simulink model "hand_nofeedback"  (R2013a)
settings: Solver=ode45  StartTime=0.0  StopTime=10.0  MaxStep=1  RelTol=1e-3
values from neighbouring files (symbols this model uses):
  m = size(t,2)    [ff.m]    (also in findGradientPend.m; interpolate.m = min(dss,[],2))
  s = @(t) [sqrt(l^2 - p(2,t).^2) + p(1,t) ; 0]    [basic.m]    (also in evaluate.m = model(p); f.m = [[l;0] zeros(2,n-1)]; ff.m = [[l;0] zeros(2,m-1)]; model.m = zeros(2,1))
libraries: mblibv1 x14, simulink x5
settings Model: Creator=annie  LastModifiedBy=simplehands
settings DataIOCC: SignalLoggingSaveFormat=ModelDataLogs
settings OptimizationCC: ExpressionDepthLimit=2147483647
settings DebuggingCC: FcnCallInpInsideContextMsg=EnableAllAsWarning
settings SimMechanicsCC: VisDuringSimulation=on

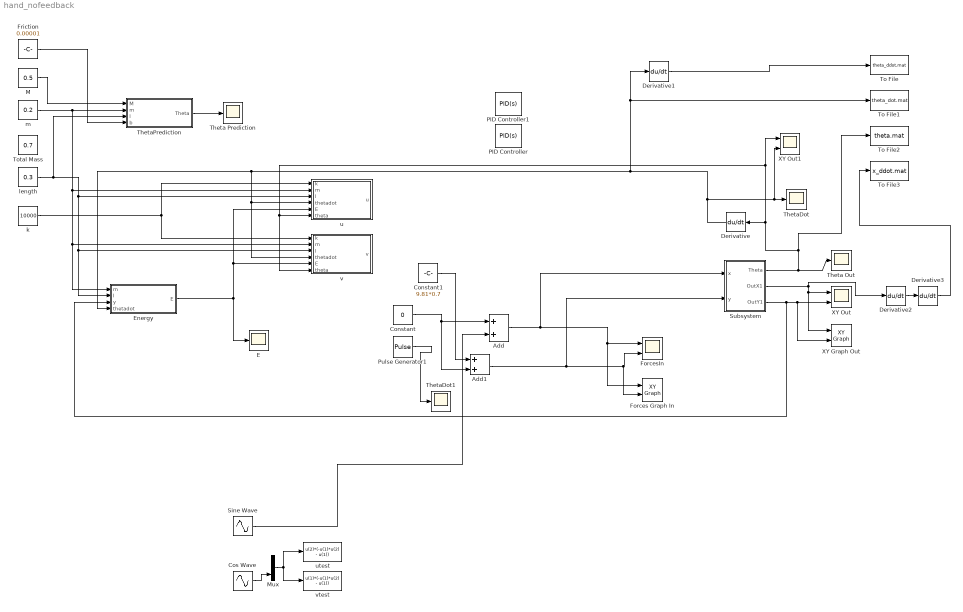
== system hand_nofeedback ==
  Add : Sum
  Add1 : Sum
  Constant : Constant  Value=0
  Constant1 : Constant  Value=9.81*0.7
  Cos Wave : Sin  Phase=pi/2  SampleTime=0
  Derivative{,1..3} (4 alike) : Derivative
  E : Scope
      settings: TimeRange=10  YMin=-0.025  YMax=0.0025  SaveName=ScopeData5
  Energy : Subsystem
  Forces Graph In : simulink/Sinks/XY Graph  xmin=-1  xmax=1  ymin=-1  ymax=1  st=-1
  ForcesIn : Scope  NumInputPorts=2
      settings: TimeRange=10  YMin=-0.1~-0.1  YMax=0.25~0.25  SaveName=ScopeData2
  Friction : Constant  Value=0.00001
  M : Constant  Value=0.5
  Mux : Mux  Inputs=2
  PID Controller : simulink/Continuous/PID Controller  Controller=PID  TimeDomain=Continuous-time  SampleTime=1  IntegratorMethod=Forward Euler  FilterMethod=Forward Euler  Form=Parallel  P=1  I=1  D=0  N=100  InitialConditionSource=internal  InitialConditionForIntegrator=0  InitialConditionForFilter=0  ExternalReset=none  LimitOutput=off  UpperSaturationLimit=inf  LowerSaturationLimit=-inf  LinearizeAsGain=on  AntiWindupMode=none  Kb=1  TrackingMode=off  Kt=1  PParamMin=[]  PParamMax=[]  IParamMin=[]  IParamMax=[]  DParamMin=[]  DParamMax=[]  NParamMin=[]  NParamMax=[]  KbParamMin=[]  KbParamMax=[]  KtParamMin=[]  KtParamMax=[]  POutMin=[]  POutMax=[]  IOutMin=[]  IOutMax=[]  DOutMin=[]  DOutMax=[]  NOutMin=[]  NOutMax=[]  KbOutMin=[]  KbOutMax=[]  KtOutMin=[]  KtOutMax=[]  IntegratorOutMin=[]  IntegratorOutMax=[]  FilterOutMin=[]  FilterOutMax=[]  SumOutMin=[]  SumOutMax=[]  SumI1OutMin=[]  SumI1OutMax=[]  SumI2OutMin=[]  SumI2OutMax=[]  SumI3OutMin=[]  SumI3OutMax=[]  SumDOutMin=[]  SumDOutMax=[]  SaturationOutMin=[]  SaturationOutMax=[]  IntegratorContinuousStateAttributes=''  IntegratorStateMustResolveToSignalObject=off  IntegratorRTWStateStorageClass=Auto  FilterContinuousStateAttributes=''  FilterStateMustResolveToSignalObject=off  FilterRTWStateStorageClass=Auto
  PID Controller1 : simulink/Continuous/PID Controller  Controller=PID  TimeDomain=Continuous-time  SampleTime=1  IntegratorMethod=Forward Euler  FilterMethod=Forward Euler  Form=Parallel  P=1  I=1  D=0  N=100  InitialConditionSource=internal  InitialConditionForIntegrator=0  InitialConditionForFilter=0  ExternalReset=none  LimitOutput=off  UpperSaturationLimit=inf  LowerSaturationLimit=-inf  LinearizeAsGain=on  AntiWindupMode=none  Kb=1  TrackingMode=off  Kt=1  PParamMin=[]  PParamMax=[]  IParamMin=[]  IParamMax=[]  DParamMin=[]  DParamMax=[]  NParamMin=[]  NParamMax=[]  KbParamMin=[]  KbParamMax=[]  KtParamMin=[]  KtParamMax=[]  POutMin=[]  POutMax=[]  IOutMin=[]  IOutMax=[]  DOutMin=[]  DOutMax=[]  NOutMin=[]  NOutMax=[]  KbOutMin=[]  KbOutMax=[]  KtOutMin=[]  KtOutMax=[]  IntegratorOutMin=[]  IntegratorOutMax=[]  FilterOutMin=[]  FilterOutMax=[]  SumOutMin=[]  SumOutMax=[]  SumI1OutMin=[]  SumI1OutMax=[]  SumI2OutMin=[]  SumI2OutMax=[]  SumI3OutMin=[]  SumI3OutMax=[]  SumDOutMin=[]  SumDOutMax=[]  SaturationOutMin=[]  SaturationOutMax=[]  IntegratorContinuousStateAttributes=''  IntegratorStateMustResolveToSignalObject=off  IntegratorRTWStateStorageClass=Auto  FilterContinuousStateAttributes=''  FilterStateMustResolveToSignalObject=off  FilterRTWStateStorageClass=Auto
  Pulse Generator1 : DiscretePulseGenerator  PulseType=Time based  Amplitude=100  Period=100  PulseWidth=0.01
  Sine Wave : Sin  Frequency=1/1.098  Phase=pi/2  SampleTime=0
  Subsystem : Subsystem
  Theta Prediction : Scope
      settings: TimeRange=10  YMin=-2  YMax=0.25
  Theta Out : Scope
      settings: YMin=-3.5  YMax=3
  ThetaDot : Scope
      settings: TimeRange=10  YMin=-0.000525  YMax=-0.00035  SaveName=ScopeData6
  ThetaDot1 : Scope
      settings: TimeRange=10  YMin=-0.025  YMax=0.0025  SaveName=ScopeData9
  ThetaPrediction : Subsystem
  To File : ToFile  Filename=theta_ddot.mat  MatrixName=theta_ddot  SaveFormat=Timeseries
  To File1 : ToFile  Filename=theta_dot.mat  MatrixName=theta_dot  SaveFormat=Timeseries
  To File2 : ToFile  Filename=theta.mat  MatrixName=theta  SaveFormat=Timeseries
  To File3 : ToFile  Filename=x_ddot.mat  MatrixName=x_ddot  SaveFormat=Timeseries
  Total Mass : Constant  Value=0.7
  XY Graph Out : simulink/Sinks/XY Graph  xmin=-1  xmax=1  ymin=-1  ymax=1  st=-1
  XY Out : Scope  NumInputPorts=2
      settings: TimeRange=10  YMin=-1~-35000  YMax=1~-25000  SaveName=ScopeData3
  XY Out1 : Scope  NumInputPorts=2
      settings: TimeRange=10  YMin=-7.5~-500  YMax=0~0  SaveName=ScopeData8
  k : Constant  Value=10000
  length : Constant  Value=0.3
  m : Constant  Value=0.2
  u : Subsystem
  utest : Fcn  Expr=u(2)*(-u(1)*u(2) - u(1))
  v : Subsystem
  vtest : Fcn  Expr=u(1)*(-u(1)*u(2) - u(1))
  wires:
  Subsystem/2(OutX1) -> XY Graph Out/1, XY Out/1, Derivative2/1
  Subsystem/3(OutY1) -> Energy/3(y), XY Graph Out/2, XY Out/2
  length/1 -> ThetaPrediction/3(l), Energy/2(l), v/3(l), u/3(l)
  Friction/1 -> ThetaPrediction/4(b)
  m/1 -> u/2(m), Energy/1(m), v/2(m), ThetaPrediction/2(m)
  M/1 -> ThetaPrediction/1(M)
  ThetaPrediction/1(Theta) -> Theta Prediction/1
  Mux/1 -> utest/1, vtest/1
  Cos Wave/1 -> Mux/2
  Derivative/1 -> XY Out1/2, ThetaDot/1, Energy/4(thetadot), v/4(thetadot), u/4(thetadot), To File1/1, Derivative1/1
  k/1 -> u/1(k), v/1(k)
  Energy/1(E) -> E/1, u/5(E), v/5(E)
  Subsystem/1(Theta) -> To File2/1, XY Out1/1, v/6(theta), u/6(theta), Derivative/1, Theta Out/1
  Add/1 -> Subsystem/1(x), Forces Graph In/1, ForcesIn/1
  Add1/1 -> Subsystem/2(y), Forces Graph In/2, ForcesIn/2
  Constant/1 -> Add1/2, Add/1
  Constant1/1 -> Add1/1
  Pulse Generator1/1 -> ThetaDot1/1
  Sine Wave/1 -> Add/2
  Derivative1/1 -> To File/1
  Derivative2/1 -> Derivative3/1
  Derivative3/1 -> To File3/1

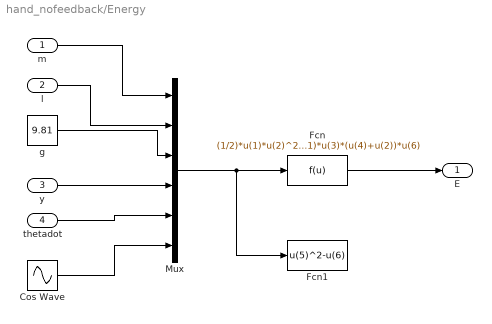
== system hand_nofeedback/Energy ==
  m : Inport
  l : Inport  Port=2
  y : Inport  Port=3
  thetadot : Inport  Port=4
  Cos Wave : Sin  Phase=pi/2  SampleTime=0
  Fcn : Fcn  Expr=(1/2)*u(1)*u(2)^2*u(5)^2 - u(1)*u(3)*(u(4)+u(2))*u(6)
  Fcn1 : Fcn  Expr=u(5)^2-u(6)
  Mux : Mux  Inputs=6
  g : Constant  Value=9.81
  E : Outport
  wires:
  m/1 -> Mux/1
  l/1 -> Mux/2
  g/1 -> Mux/3
  Cos Wave/1 -> Mux/6
  Mux/1 -> Fcn1/1, Fcn/1
  thetadot/1 -> Mux/5
  y/1 -> Mux/4
  Fcn/1 -> E/1

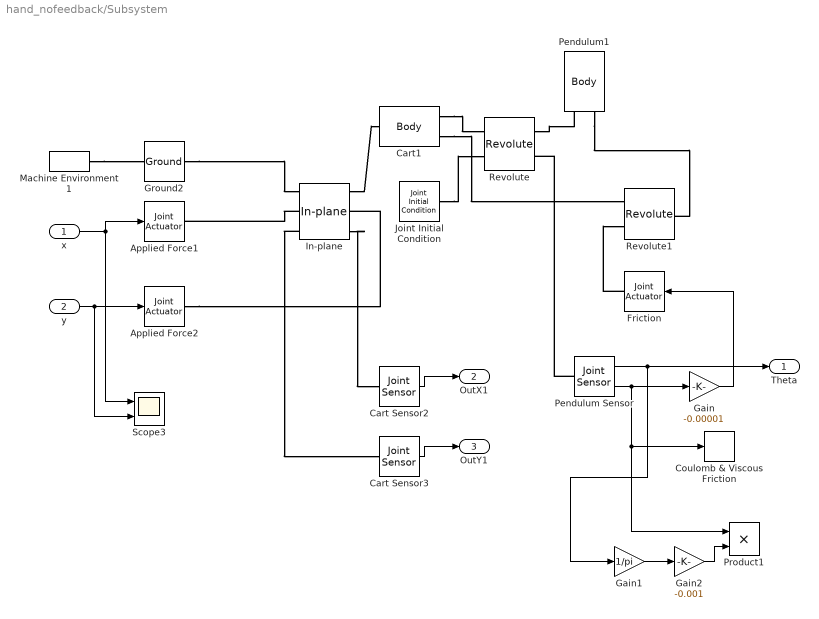
== system hand_nofeedback/Subsystem ==
  x : Inport
  y : Inport  Port=2
  Applied Force1 : mblibv1/Sensors &  Actuators/Joint Actuator  UpdateFromCAD=off  PhysicalDomain=Mechanical  PortType=blob  ActuationStyle=Force  AngleUnits=deg  ArcVelocityUnits=deg/s  ArcAccelerationUnits=deg/s^2  CoordPositionUnits=m  VelocityUnits=m/s  AccelerationUnits=m/s^2  ForceUnits=N  TorqueUnits=N*m  ActiveIO=on  Width=1  DialogClass=MechanicalActuatorBlock  Primitive=P1  ReferenceFrame=Absolute (World)
  Applied Force2 : mblibv1/Sensors &  Actuators/Joint Actuator  UpdateFromCAD=off  PhysicalDomain=Mechanical  PortType=blob  ActuationStyle=Force  AngleUnits=deg  ArcVelocityUnits=deg/s  ArcAccelerationUnits=deg/s^2  CoordPositionUnits=m  VelocityUnits=m/s  AccelerationUnits=m/s^2  ForceUnits=N  TorqueUnits=N*m  ActiveIO=on  Width=1  DialogClass=MechanicalActuatorBlock  Primitive=P2  ReferenceFrame=Absolute (World)
  Cart Sensor2 : mblibv1/Sensors &  Actuators/Joint Sensor  UpdateFromCAD=off  PhysicalDomain=Mechanical  PortType=blob  Muxed=off  Pose=off  Angle=on  AngleUnits=deg  ArcVelocity=off  ArcVelocityUnits=deg/s  ArcAcceleration=off  ArcAccelerationUnits=deg/s^2  CoordPosition=on  CoordPositionUnits=m  Velocity=off  VelocityUnits=m/s  Acceleration=off  AccelerationUnits=m/s^2  Quaternion=on  QuaternionDT=off  QuaternionDDT=off  QuaternionUnits=off  OutputVector=[1]  ActiveIO=on  Width=1  DialogClass=MechanicalSensorBlock  Primitive=P1  Force=off  ForceUnits=N  Torque=off  TorqueUnits=N*m  ReferenceFrame=Absolute (World)  ReactionSensedSide=Base  ReactionReferenceFrame=Absolute (World)  ReactionForce=off  ReactionForceUnits=N  ReactionMoment=off  ReactionMomentUnits=N*m
  Cart Sensor3 : mblibv1/Sensors &  Actuators/Joint Sensor  UpdateFromCAD=off  PhysicalDomain=Mechanical  PortType=blob  Muxed=off  Pose=off  Angle=on  AngleUnits=deg  ArcVelocity=off  ArcVelocityUnits=deg/s  ArcAcceleration=off  ArcAccelerationUnits=deg/s^2  CoordPosition=on  CoordPositionUnits=m  Velocity=off  VelocityUnits=m/s  Acceleration=off  AccelerationUnits=m/s^2  Quaternion=on  QuaternionDT=off  QuaternionDDT=off  QuaternionUnits=off  OutputVector=[1]  ActiveIO=on  Width=1  DialogClass=MechanicalSensorBlock  Primitive=P2  Force=off  ForceUnits=N  Torque=off  TorqueUnits=N*m  ReferenceFrame=Absolute (World)  ReactionSensedSide=Base  ReactionReferenceFrame=Absolute (World)  ReactionForce=off  ReactionForceUnits=N  ReactionMoment=off  ReactionMomentUnits=N*m
  Cart1 : mblibv1/Bodies/Body  LConnTagsString=CS1  RConnTagsString=CS2|CS3  UpdateFromCAD=off  DialogClass=MechanicalBodyBlock  Mass=0.5  MassUnits=kg  InertiaUnits=kg*m^2  Inertia=eye(3)  Shape=Cylinder  ShapeDims=[1 1]  ShapeUnits=m  ShapeUse=false  Density=1  DensityUnits=kg/m^3  DensityUse=false  GraphicsMode=MACHINE_DEFAULT  BodyColorSelMode=MACHINE_DEFAULT  BodyColor=[1 0 0]  AttachedToCS=CG  CG=Left$CG$[0 0 0]$WORLD$WORLD$m$[0 0 0]$Euler X-Y-Z$deg$WORLD$false$none  WorkingFrames=Right$CS2$[0 0.5 0]$CG$CG$m$[0 0 0]$Euler X-Y-Z$deg$WORLD$true$none#Left$CS1$[0 0 0]$CG$CG$m$[0 0 0]$Euler X-Y-Z$deg$WORLD$true$none#Right$CS3$[0 0.5 0]$CG$CG$m$[0 0 0]$Euler X-Y-Z$deg$WORLD$true$none#Left$CS4$[0 0 0]$CG$CG$m$[0 0 0]$Euler X-Y-Z$deg$WORLD$false$none#Left$CS8$[-1 0.5 0]$CG$CG$m$[0 0 0]$Euler X-Y-Z$deg$WORLD$false$none#Right$CS5$[-1 -0.5 0]$CG$CG$m$[0 0 0]$Euler X-Y-Z$deg$WORLD$false$none#Right$CS6$[1 -0.5 0]$CG$CG$m$[0 0 0]$Euler X-Y-Z$deg$WORLD$false$none#Right$CS7$[1 0.5 0]$CG$CG$m$[0 0 0]$Euler X-Y-Z$deg$WORLD$false$none  CGPos=[0 0 0]  CGRot=[0 0 0]  CS0Pos=[]  CS0Rot=[]  CS1Pos=[0 0 0]  CS1Rot=[0 0 0]  CS2Pos=[0 0.5 0]  CS2Rot=[0 0 0]  CS3Pos=[0 0.5 0]  CS3Rot=[0 0 0]  CS4Pos=[0 0 0]  CS4Rot=[0 0 0]  CS5Pos=[-1 -0.5 0]  CS5Rot=[0 0 0]  CS6Pos=[1 -0.5 0]  CS6Rot=[0 0 0]  CS7Pos=[1 0.5 0]  CS7Rot=[0 0 0]  CS8Pos=[-1 0.5 0]  CS8Rot=[0 0 0]  CS9Pos=[]  CS9Rot=[]  CS10Pos=[]  CS10Rot=[]  CS11Pos=[]  CS11Rot=[]  CS12Pos=[]  CS12Rot=[]  CS13Pos=[]  CS13Rot=[]  CS14Pos=[]  CS14Rot=[]  CS15Pos=[]  CS15Rot=[]  CS16Pos=[]  CS16Rot=[]  CS17Pos=[]  CS17Rot=[]  CS18Pos=[]  CS18Rot=[]  CS19Pos=[]  CS19Rot=[]  CS20Pos=[]  CS20Rot=[]
  Coulomb & Viscous Friction : simulink/Discontinuities/Coulomb & Viscous Friction  offset=-0.01  gain=0.00001
  Friction : mblibv1/Sensors &  Actuators/Joint Actuator  UpdateFromCAD=off  PhysicalDomain=Mechanical  PortType=blob  ActuationStyle=Force  AngleUnits=deg  ArcVelocityUnits=deg/s  ArcAccelerationUnits=deg/s^2  CoordPositionUnits=m  VelocityUnits=m/s  AccelerationUnits=m/s^2  ForceUnits=N  TorqueUnits=N*m  ActiveIO=on  Width=1  DialogClass=MechanicalActuatorBlock  Primitive=R1  ReferenceFrame=Absolute (World)
  Gain : Gain  Gain=-0.00001
  Gain1 : Gain  Gain=1/pi
  Gain2 : Gain  Gain=-0.001
  Ground2 : mblibv1/Bodies/Ground  UpdateFromCAD=off  LeftPortType=env  RightPortType=workingframe  PhysicalDomain=Mechanical  DialogClass=GroundBlock  CoordPosition=[0 0 0]  CoordPositionUnits=m  StateVectorMgrId=0  MachineId=[1 0]  ShowEnvPort=on
  In-plane : mblibv1/Joints/In-plane  LConnTagsString=__newl0|SA1|SA2  RConnTagsString=__newr0|SA1|SA2  UpdateFromCAD=off  NumSAPorts=4  CutJoint=off  MarkAsCut=off  Primitives=prismatic  PrimitiveProps=P1$World$[1 0 0]$prismatic#P2$World$[0 1 0]$prismatic  DialogClass=JointBlock  P1Axis=[1 0 0]  P2Axis=[0 1 0]
  Joint Initial Condition : mblibv1/Sensors &  Actuators/Joint Initial Condition  UpdateFromCAD=off  LeftPortType=blob  RightPortType=blob  PhysicalDomain=mechanical  DialogClass=InitialConditionBlock  InitialConditions=P1$false$0$m$deg$0$m/s$deg/s#P2$false$0$m$deg$0$m/s$deg/s#P3$false$0$m$deg$0$m/s$deg/s#R1$true$0$m$rad$0$m/s$deg/s#R2$false$0$m$deg$0$m/s$deg/s#R3$false$0$m$deg$0$m/s$deg/s#S$false$0$m$deg$0$m/s$deg/s  P1PIC=0  P1VIC=0  P2PIC=0  P2VIC=0  P3PIC=0  P3VIC=0  R1PIC=0  R1VIC=0  R2PIC=0  R2VIC=0  R3PIC=0  R3VIC=0  SPIC=0  SVIC=0
  Machine Environment1 : mblibv1/Bodies/Machine Environment  PortType=env  PhysicalDomain=Mechanical  DialogTemplateClass=MECH.MachineEnvironment  SyncWhenCopied=off  Gravity=[0 -9.81 0]  GravityUnits=m/s^2  GravityAsSignal=off  Dimensionality=Auto-detect  AnalysisType=Forward dynamics  LinearAssemblyTolerance=1e-3  LinearAssemblyToleranceUnits=m  AngularAssemblyTolerance=1e-3  AngularAssemblyToleranceUnits=rad  ConstraintSolverType=Stabilizing  ConstraintRelTolerance=1e-4  ConstraintAbsTolerance=1e-4  UseRobustSingularityHandling=off  RedundancyAnalysisToleranceType=Automatically select tolerance  RedundancyAnalysisTolerance=1e-14  StatePerturbationType=Fixed  PerturbationSize=1e-5  VisualizeMachine=on  BodyVisualizationType=Use model default body geometries  BodyColorSelMode=Use model default  DefaultBodyColor=[1 0 0]
  Pendulum Sensor : mblibv1/Sensors &  Actuators/Joint Sensor  UpdateFromCAD=off  PhysicalDomain=Mechanical  PortType=blob  Muxed=off  Pose=off  Angle=on  AngleUnits=rad  ArcVelocity=on  ArcVelocityUnits=deg/s  ArcAcceleration=off  ArcAccelerationUnits=deg/s^2  CoordPosition=on  CoordPositionUnits=m  Velocity=off  VelocityUnits=m/s  Acceleration=off  AccelerationUnits=m/s^2  Quaternion=on  QuaternionDT=off  QuaternionDDT=off  QuaternionUnits=off  OutputVector=[1]  ActiveIO=on  Width=2  DialogClass=MechanicalSensorBlock  Primitive=R1  Force=off  ForceUnits=N  Torque=off  TorqueUnits=N*m  ReferenceFrame=Absolute (World)  ReactionSensedSide=Base  ReactionReferenceFrame=Absolute (World)  ReactionForce=off  ReactionForceUnits=N  ReactionMoment=off  ReactionMomentUnits=N*m
  Pendulum1 : mblibv1/Bodies/Body  LConnTagsString=CS6|CS1  UpdateFromCAD=off  DialogClass=MechanicalBodyBlock  Mass=0.2  MassUnits=kg  InertiaUnits=kg*m^2  Inertia=0.006*eye(3)  Shape=Cylinder  ShapeDims=[1 1]  ShapeUnits=m  ShapeUse=false  Density=1  DensityUnits=kg/m^3  DensityUse=false  GraphicsMode=MACHINE_DEFAULT  BodyColorSelMode=COLORPALETTE  BodyColor=[0.078431 0.16863 0.54902]  AttachedToCS=CG  CG=Left$CG$[0 -0.3 0]$CS1$CS1$m$[0 0 0]$Euler X-Y-Z$deg$WORLD$false$none  WorkingFrames=Left$CS6$[0 0 0]$Adjoining$Adjoining$m$[0 0 0]$Euler X-Y-Z$deg$WORLD$true$none#Left$CS1$[0 0 0]$Adjoining$Adjoining$m$[0 0 0]$Euler X-Y-Z$deg$WORLD$true$none#Right$CS2$[0.1 0 0]$CS1$CS1$m$[0 0 0]$Euler X-Y-Z$deg$WORLD$false$none#Right$CS3$[-0.1 0 0]$CS1$CS1$m$[0 0 0]$Euler X-Y-Z$deg$WORLD$false$none#Right$CS4$[-0.1 -0.6 0]$CS1$CS1$m$[0 0 0]$Euler X-Y-Z$deg$WORLD$false$none#Right$CS5$[0.1 -0.6 0]$CS1$CS1$m$[0 0 0]$Euler X-Y-Z$deg$WORLD$false$none  CGPos=[0 -0.3 0]  CGRot=[0 0 0]  CS0Pos=[]  CS0Rot=[]  CS1Pos=[0 0 0]  CS1Rot=[0 0 0]  CS2Pos=[0.1 0 0]  CS2Rot=[0 0 0]  CS3Pos=[-0.1 0 0]  CS3Rot=[0 0 0]  CS4Pos=[-0.1 -0.6 0]  CS4Rot=[0 0 0]  CS5Pos=[0.1 -0.6 0]  CS5Rot=[0 0 0]  CS6Pos=[0 0 0]  CS6Rot=[0 0 0]  CS7Pos=[]  CS7Rot=[]  CS8Pos=[]  CS8Rot=[]  CS9Pos=[]  CS9Rot=[]  CS10Pos=[]  CS10Rot=[]  CS11Pos=[]  CS11Rot=[]  CS12Pos=[]  CS12Rot=[]  CS13Pos=[]  CS13Rot=[]  CS14Pos=[]  CS14Rot=[]  CS15Pos=[]  CS15Rot=[]  CS16Pos=[]  CS16Rot=[]  CS17Pos=[]  CS17Rot=[]  CS18Pos=[]  CS18Rot=[]  CS19Pos=[]  CS19Rot=[]  CS20Pos=[]  CS20Rot=[]
  Product1 : Product
  Revolute : mblibv1/Joints/Revolute  LConnTagsString=__newl0|SA1  RConnTagsString=__newr0|SA1  UpdateFromCAD=off  NumSAPorts=2  CutJoint=off  MarkAsCut=off  Primitives=prismatic  PrimitiveProps=R1$World$[0 0 1]$revolute  DialogClass=JointBlock  R1Axis=[0 0 1]
  Revolute1 : mblibv1/Joints/Revolute  LConnTagsString=__newl0|SA1  RConnTagsString=__newr0  UpdateFromCAD=off  NumSAPorts=1  CutJoint=off  MarkAsCut=off  Primitives=prismatic  PrimitiveProps=R1$World$[0 0 1]$revolute  DialogClass=JointBlock  R1Axis=[0 0 1]
  Scope3 : Scope  NumInputPorts=2
      settings: TimeRange=10  YMin=-500~-300  YMax=2500~300  SaveName=ScopeData4
  Theta : Outport
  OutX1 : Outport  Port=2
  OutY1 : Outport  Port=3
  wires:
  x/1 -> Scope3/1, Applied Force1/1
  Cart Sensor2/1 -> OutX1/1
  Cart Sensor3/1 -> OutY1/1
  y/1 -> Scope3/2, Applied Force2/1
  Pendulum Sensor/2 -> Gain/1, Coulomb & Viscous Friction/1, Product1/1
  Gain1/1 -> Gain2/1
  Gain2/1 -> Product1/2
  Pendulum Sensor/1 -> Gain1/1, Theta/1
  Gain/1 -> Friction/1
  connections:
  Joint Initial Condition/RConn1 -- Revolute/LConn2
  In-plane/RConn1 -- Cart1/LConn1
  Machine Environment1/RConn1 -- Ground2/LConn1
  Ground2/RConn1 -- In-plane/LConn1
  In-plane/LConn2 -- Applied Force1/RConn1
  Pendulum Sensor/LConn1 -- Revolute/RConn2
  Applied Force2/RConn1 -- In-plane/RConn2
  In-plane/LConn3 -- Cart Sensor3/LConn1
  In-plane/RConn3 -- Cart Sensor2/LConn1
  Cart1/RConn1 -- Revolute/LConn1
  Cart1/RConn2 -- Revolute1/LConn1
  Revolute/RConn1 -- Pendulum1/LConn1
  Pendulum1/LConn2 -- Revolute1/RConn1
  Friction/RConn1 -- Revolute1/LConn2

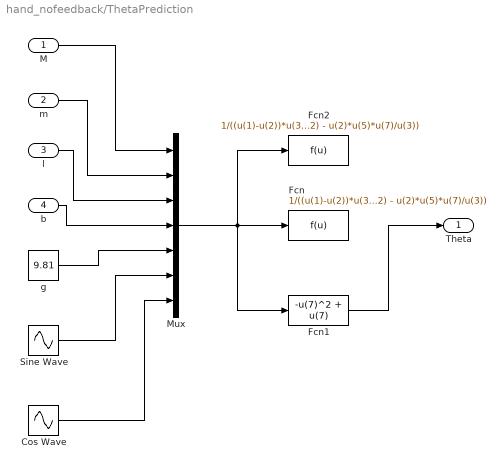
== system hand_nofeedback/ThetaPrediction ==
  M : Inport
  m : Inport  Port=2
  l : Inport  Port=3
  b : Inport  Port=4
  Cos Wave : Sin  Phase=pi/2  SampleTime=0
  Fcn : Fcn  Expr=1/((u(1)-u(2))*u(3) + (u(4)/u(3))) * (((-1/2)*u(2)*u(5)*u(7)^2) - u(2)*u(5)*u(7)/u(3))
  Fcn1 : Fcn  Expr=-u(7)^2 + u(7)
  Fcn2 : Fcn  Expr=1/((u(1)-u(2))*u(3)) * (((-1/2)*u(2)*u(5)*u(7)^2) - u(2)*u(5)*u(7)/u(3))
  Mux : Mux  Inputs=7
  Sine Wave : Sin  SampleTime=0
  g : Constant  Value=9.81
  Theta : Outport
  wires:
  M/1 -> Mux/1
  m/1 -> Mux/2
  l/1 -> Mux/3
  b/1 -> Mux/4
  g/1 -> Mux/5
  Sine Wave/1 -> Mux/6
  Cos Wave/1 -> Mux/7
  Mux/1 -> Fcn1/1, Fcn2/1, Fcn/1
  Fcn1/1 -> Theta/1

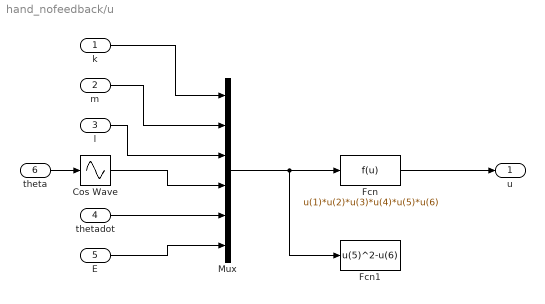
== system hand_nofeedback/u ==
  k : Inport
  m : Inport  Port=2
  l : Inport  Port=3
  thetadot : Inport  Port=4
  E : Inport  Port=5
  theta : Inport  Port=6
  Cos Wave : Sin  TimeSource=Use external signal  Phase=pi/2  SampleTime=0
  Fcn : Fcn  Expr=u(1)*u(2)*u(3)*u(4)*u(5)*u(6)
  Fcn1 : Fcn  Expr=u(5)^2-u(6)
  Mux : Mux  Inputs=6
  u : Outport
  wires:
  k/1 -> Mux/1
  m/1 -> Mux/2
  Cos Wave/1 -> Mux/4
  Mux/1 -> Fcn1/1, Fcn/1
  thetadot/1 -> Mux/5
  l/1 -> Mux/3
  Fcn/1 -> u/1
  E/1 -> Mux/6
  theta/1 -> Cos Wave/1

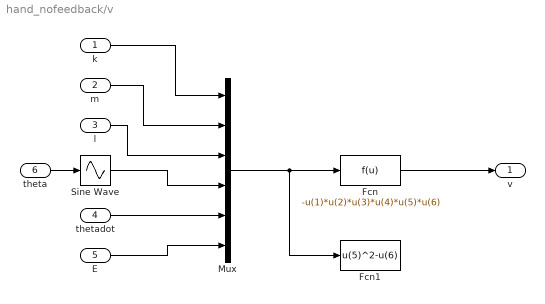
== system hand_nofeedback/v ==
  k : Inport
  m : Inport  Port=2
  l : Inport  Port=3
  thetadot : Inport  Port=4
  E : Inport  Port=5
  theta : Inport  Port=6
  Fcn : Fcn  Expr=-u(1)*u(2)*u(3)*u(4)*u(5)*u(6)
  Fcn1 : Fcn  Expr=u(5)^2-u(6)
  Mux : Mux  Inputs=6
  Sine Wave : Sin  TimeSource=Use external signal  SampleTime=0
  v : Outport
  wires:
  k/1 -> Mux/1
  m/1 -> Mux/2
  Sine Wave/1 -> Mux/4
  Mux/1 -> Fcn1/1, Fcn/1
  thetadot/1 -> Mux/5
  l/1 -> Mux/3
  Fcn/1 -> v/1
  E/1 -> Mux/6
  theta/1 -> Sine Wave/1
